simulink model "FOPIDSOCOptimRand"  (R2019b)
settings: Solver=FixedStepAuto  StartTime=0.0  StopTime=30000  FixedStep=0.01  RelTol=1e-3
values from neighbouring files (symbols this model uses):
  L = 10    [benchmarkFOPIDStartReal.m]    (also in benchmarkFOPIStartRealIOLoopL01FOG.m = 0.1; benchmarkFOPIStartRealIOLoopL10FOG.m; benchmarkFOPIStartRealIOLoopL1FOG.m = 1)
  lambdaO = 0.8    [benchmarkFOPIStartRealIOLoopL01FOG.m]
  maxKi = 0.1    [benchmarkFOPIDStartReal.m]    (also in benchmarkFOPIStartRealIOLoopL01FOG.m = 1; benchmarkFOPIStartRealIOLoopL10FOG.m = 0.6; benchmarkFOPIStartRealIOLoopL1FOG.m = 1)
  maxKp = 0.1    [benchmarkFOPIDStartReal.m]    (also in benchmarkFOPIStartRealIOLoopL01FOG.m = 3; benchmarkFOPIStartRealIOLoopL10FOG.m = 2; benchmarkFOPIStartRealIOLoopL1FOG.m = 2)
  minKi = 0.001    [benchmarkFOPIDStartReal.m]    (also in benchmarkFOPIStartRealIOLoopL01FOG.m = 0.3; benchmarkFOPIStartRealIOLoopL10FOG.m = 0.2; benchmarkFOPIStartRealIOLoopL1FOG.m = 0.3)
  minKp = 0.01    [benchmarkFOPIDStartReal.m]    (also in benchmarkFOPIStartRealIOLoopL01FOG.m = 0.3; benchmarkFOPIStartRealIOLoopL10FOG.m = 0.3; benchmarkFOPIStartRealIOLoopL1FOG.m = 0.3)
  ts = 0.01    [benchmarkFOPIStartRealIOLoopL01FOG.m]    (also in benchmarkFOPIStartRealIOLoopL10FOG.m; benchmarkFOPIStartRealIOLoopL1FOG.m; settlingTime.m = time(end))
libraries: dspmathops x1
settings Model: Creator=jairo  LastModifiedBy=jairo
settings DataIOCC: ReturnWorkspaceOutputs=off
settings DebuggingCC: ArithmeticOperatorsInVariantConditions=warning
settings SFSimCC: CustomCodeUndefinedFunction=UseInterfaceOnly

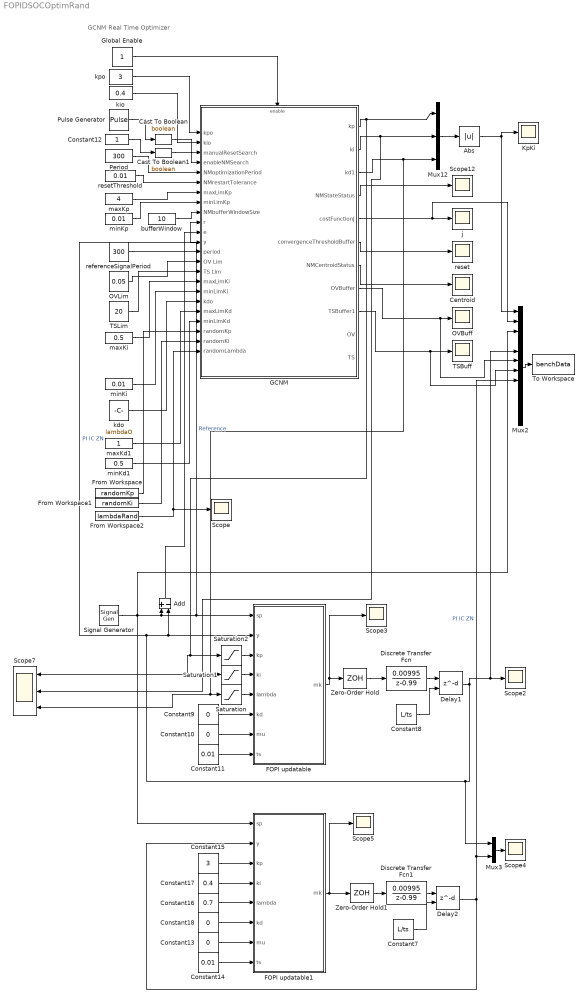
== system FOPIDSOCOptimRand ==
  note: GCNM Real Time Optimizer
  Abs : Abs
  Add : Sum  Inputs=+-
  Cast To Boolean : DataTypeConversion  OutDataTypeStr=boolean
  Cast To Boolean1 : DataTypeConversion  OutDataTypeStr=boolean
  Centroid : Scope
  Constant{9..10,13,18} (4 alike) : Constant  Value=0
  Constant11 : Constant  Value=0.01
  Constant12 : Constant  OutDataTypeStr=boolean
  Constant14 : Constant  Value=0.01
  Constant15 : Constant  Value=3
  Constant16 : Constant  Value=0.7
  Constant17 : Constant  Value=0.4
  Constant7 : Constant  Value=L/ts
  Constant8 : Constant  Value=L/ts
  Delay1 : Delay  DelayLengthSource=Input port
      settings: InputPortMap=u0,p1
  Delay2 : Delay  DelayLengthSource=Input port
      settings: InputPortMap=u0,p1
  Discrete Transfer Fcn : DiscreteTransferFcn  Numerator=[0.00995]  Denominator=[1 -0.99]
  Discrete Transfer Fcn1 : DiscreteTransferFcn  Numerator=[0.00995]  Denominator=[1 -0.99]
  FOPI updatable : Stateflow chart  TreatAsAtomicUnit=on
  FOPI updatable1 : Stateflow chart  TreatAsAtomicUnit=on
  From Workspace : FromWorkspace  VariableName=randomKp  SampleTime=0
  From Workspace1 : FromWorkspace  VariableName=randomKi  SampleTime=0
  From Workspace2 : FromWorkspace  VariableName=lambdaRand  SampleTime=0
  GCNM : Subsystem
  Global Enable : Constant
  KpKi : Scope
  Mux12 : Mux  Inputs=3
  Mux2 : Mux  Inputs=12
  Mux3 : Mux  Inputs=2
  OVBuff : Scope
  OVLim : Constant  Value=0.05
  Period : Constant  Value=300  OutDataTypeStr=double
  Pulse Generator : DiscretePulseGenerator  PulseType=Time based  Period=20  PulseWidth=0.1
  Saturation : Saturate  UpperLimit=1  LowerLimit=0.7
  Saturation1 : Saturate  UpperLimit=maxKi  LowerLimit=minKi
  Saturation2 : Saturate  UpperLimit=maxKp  LowerLimit=minKp
  Scope{,2..5,12} (6 alike) : Scope
  Scope7 : Scope  NumInputPorts=3
  Signal Generator : SignalGenerator  WaveForm=square  Frequency=1/300
  TSBuff : Scope
  TSLim : Constant  Value=20
  To Workspace : ToWorkspace  VariableName=benchData  SaveFormat=Timeseries  SampleTime=-1
  Zero-Order Hold : ZeroOrderHold  SampleTime=-1
  Zero-Order Hold1 : ZeroOrderHold  SampleTime=-1
  bufferWindow : Constant  Value=10  OutDataTypeStr=uint16
  j : Scope
  kdo : Constant  Value=lambdaO
  kio : Constant  Value=0.4  OutDataTypeStr=double
  kpo : Constant  Value=3  OutDataTypeStr=double
  maxKd1 : Constant  VectorParams1D=off  OutDataTypeStr=double
  maxKi : Constant  Value=0.5  VectorParams1D=off  OutDataTypeStr=double
  maxKp : Constant  Value=4  OutDataTypeStr=double
  minKd1 : Constant  Value=0.5  OutDataTypeStr=double
  minKi : Constant  Value=0.01  OutDataTypeStr=double
  minKp : Constant  Value=0.01  OutDataTypeStr=double
  referenceSignalPeriod : Constant  Value=300
  reset : Scope
  resetThreshold : Constant  Value=0.01
  wires:
  FOPI updatable/1(mk) -> Scope3/1, Zero-Order Hold/1
  Discrete Transfer Fcn/1 -> Delay1/1
  Constant9/1 -> FOPI updatable/6(kd)
  Constant11/1 -> FOPI updatable/8(ts)
  Constant10/1 -> FOPI updatable/7(mu)
  Delay1/1 -> Mux2/5, Scope2/1, Mux3/1, FOPI updatable/2(y), Add/2, GCNM/12("  y")  "PI IC ZN"
  maxKd1/1 -> GCNM/19(maxLimKd)
  minKd1/1 -> GCNM/20(minLimKd)
  TSLim/1 -> GCNM/15(TS Lim)
  Period/1 -> GCNM/5(NMoptimizationPeriod)
  Mux12/1 -> Abs/1
  minKi/1 -> GCNM/17(minLimKi)
  GCNM/1("  kp") -> Mux12/1, Saturation2/1, Scope7/1
  GCNM/6(convergenceThresholdBuffer) -> reset/1
  Global Enable/1 -> GCNM/Enable
  GCNM/7(NMCentroidStatus) -> Centroid/1
  Cast To Boolean1/1 -> GCNM/4(enableNMSearch)
  Mux2/1 -> To Workspace/1
  GCNM/5(costFunctionJ) -> Mux2/2, j/1
  OVLim/1 -> GCNM/14("  OV Lim")
  referenceSignalPeriod/1 -> GCNM/13("  period")
  kpo/1 -> GCNM/1(kpo)
  kdo/1 -> GCNM/18(kdo)
  maxKp/1 -> GCNM/7(maxLimKp)
  GCNM/3("  kd1") -> Saturation/1, Scope7/3, Mux12/3
  minKp/1 -> GCNM/8(minLimKp)
  GCNM/8(OVBuffer) -> Mux2/6, OVBuff/1
  Constant12/1 -> Cast To Boolean1/1
  Cast To Boolean/1 -> GCNM/3(manualResetSearch)
  maxKi/1 -> GCNM/16(maxLimKi)
  GCNM/4(NMStateStatus) -> Scope12/1
  kio/1 -> GCNM/2(kio)
  bufferWindow/1 -> GCNM/9(NMbufferWindowSize)
  GCNM/9(TSBuffer1) -> Mux2/7, TSBuff/1
  Pulse Generator/1 -> Cast To Boolean/1
  resetThreshold/1 -> GCNM/6(NMrestartTolerance)
  Signal Generator/1 -> Mux2/3, FOPI updatable1/1(sp), GCNM/10("  r"), FOPI updatable/1(sp), Add/1  "Reference"
  Add/1 -> GCNM/11("  e")
  Constant18/1 -> FOPI updatable1/6(kd)
  Constant14/1 -> FOPI updatable1/8(ts)
  Constant13/1 -> FOPI updatable1/7(mu)
  Mux3/1 -> Scope4/1
  Delay2/1 -> Mux2/8, Mux3/2, FOPI updatable1/2(y)  "PI IC ZN"
  FOPI updatable1/1(mk) -> Scope5/1, Zero-Order Hold1/1
  Constant15/1 -> FOPI updatable1/3(kp)
  Constant17/1 -> FOPI updatable1/4(ki)
  Constant16/1 -> FOPI updatable1/5(lambda)
  From Workspace/1 -> GCNM/21(randomKp)
  From Workspace1/1 -> GCNM/22(randomKi)
  From Workspace2/1 -> Scope/1, GCNM/23(randomLambda)
  Zero-Order Hold/1 -> Discrete Transfer Fcn/1
  Abs/1 -> Mux2/1, KpKi/1
  Zero-Order Hold1/1 -> Discrete Transfer Fcn1/1
  Discrete Transfer Fcn1/1 -> Delay2/1
  GCNM/2("  ki") -> Saturation1/1, Scope7/2, Mux12/2
  Saturation/1 -> FOPI updatable/5(lambda)
  Saturation1/1 -> FOPI updatable/4(ki)
  Saturation2/1 -> FOPI updatable/3(kp)
  Constant8/1 -> Delay1/2
  Constant7/1 -> Delay2/2

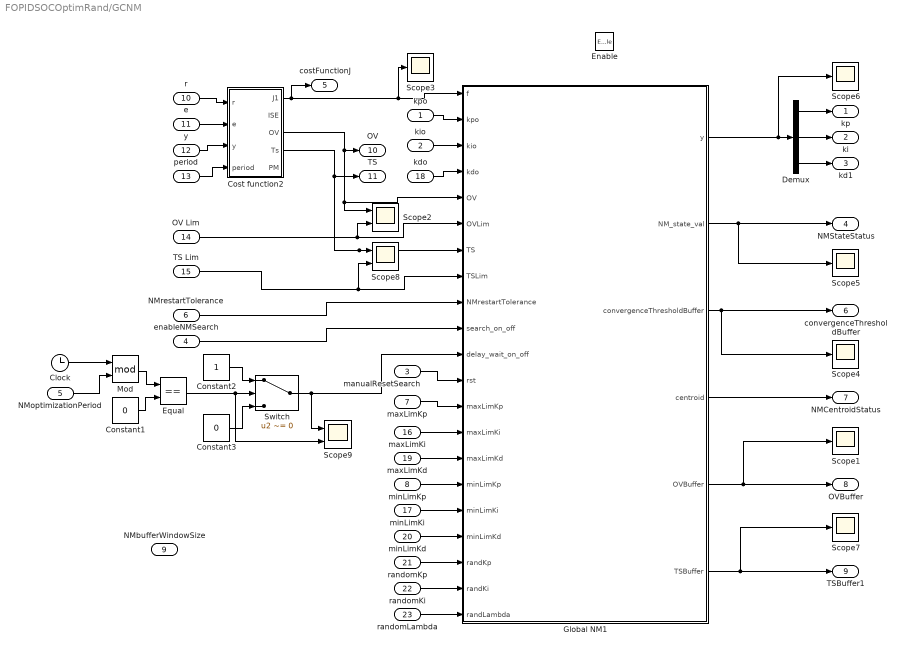
== system FOPIDSOCOptimRand/GCNM ==
  kpo : Inport  OutDataTypeStr=double
  kio : Inport  Port=2  OutDataTypeStr=double
  manualResetSearch : Inport  Port=3  OutDataTypeStr=boolean
  enableNMSearch : Inport  Port=4  OutDataTypeStr=boolean
  NMoptimizationPeriod : Inport  Port=5  OutDataTypeStr=double
  NMrestartTolerance : Inport  Port=6
  maxLimKp : Inport  Port=7  OutDataTypeStr=double
  minLimKp : Inport  Port=8  OutDataTypeStr=double
  NMbufferWindowSize : Inport  Port=9  OutDataTypeStr=uint16
  "  r" : Inport  Port=10  OutDataTypeStr=double
  "  e" : Inport  Port=11  OutDataTypeStr=double
  "  y" : Inport  Port=12  OutDataTypeStr=double
  "  period" : Inport  Port=13  OutDataTypeStr=double
  "  OV Lim" : Inport  Port=14  OutDataTypeStr=double
  TS Lim : Inport  Port=15  OutDataTypeStr=double
  maxLimKi : Inport  Port=16  OutDataTypeStr=double
  minLimKi : Inport  Port=17  OutDataTypeStr=double
  kdo : Inport  Port=18  OutDataTypeStr=double
  maxLimKd : Inport  Port=19  OutDataTypeStr=double
  minLimKd : Inport  Port=20  OutDataTypeStr=double
  randomKp : Inport  Port=21
  randomKi : Inport  Port=22
  randomLambda : Inport  Port=23
  Enable : EnablePort
  Clock : Clock
  Constant1 : Constant  Value=0
  Constant2 : Constant
  Constant3 : Constant  Value=0
  Cost function2 : Subsystem
  Demux : Demux  Outputs=3
  Equal : RelationalOperator  Operator===  RndMeth=Simplest
  Global NM1 : MATLAB Function  TreatAsAtomicUnit=on
  Mod : Math  Operator=mod  SignedPower=off  SaturateOnIntegerOverflow=on
  Scope{1,3..7} (6 alike) : Scope
  Scope2 : Scope  NumInputPorts=2
  Scope8 : Scope  NumInputPorts=2
  Scope9 : Scope  NumInputPorts=2
  Switch : Switch  Criteria=u2 ~= 0
  "  kp" : Outport  OutDataTypeStr=double
  "  ki" : Outport  Port=2  OutDataTypeStr=double
  "  kd1" : Outport  Port=3  OutDataTypeStr=double
  NMStateStatus : Outport  Port=4  OutDataTypeStr=double
  costFunctionJ : Outport  Port=5  OutDataTypeStr=double
  convergenceThresholdBuffer : Outport  Port=6  OutDataTypeStr=double
  NMCentroidStatus : Outport  Port=7  OutDataTypeStr=double
  OVBuffer : Outport  Port=8  OutDataTypeStr=double
  TSBuffer1 : Outport  Port=9  OutDataTypeStr=double
  OV : Outport  Port=10  OutDataTypeStr=double
  TS : Outport  Port=11  OutDataTypeStr=double
  wires:
  Demux/2 -> "  ki"/1
  Demux/1 -> "  kp"/1
  NMrestartTolerance/1 -> Global NM1/9(NMrestartTolerance)
  manualResetSearch/1 -> Global NM1/12(rst)
  enableNMSearch/1 -> Global NM1/10(search_on_off)
  minLimKp/1 -> Global NM1/16(minLimKp)
  maxLimKp/1 -> Global NM1/13(maxLimKp)
  Global NM1/2(NM_state_val) -> NMStateStatus/1, Scope5/1
  Global NM1/3(convergenceThresholdBuffer) -> convergenceThresholdBuffer/1, Scope4/1
  Global NM1/4(centroid) -> NMCentroidStatus/1
  Global NM1/1(y) -> Scope6/1, Demux/1
  kpo/1 -> Global NM1/2(kpo)
  kio/1 -> Global NM1/3(kio)
  Cost function2/3(OV) -> OV/1, Global NM1/5(OV), Scope2/1
  "  y"/1 -> Cost function2/3(y)
  "  e"/1 -> Cost function2/2(e)
  "  r"/1 -> Cost function2/1(r)
  Global NM1/5(OVBuffer) -> Scope1/1, OVBuffer/1
  "  period"/1 -> Cost function2/4(period)
  "  OV Lim"/1 -> Scope2/2, Global NM1/6(OVLim)
  Cost function2/4(Ts) -> TS/1, Global NM1/7(TS), Scope8/1
  TS Lim/1 -> Scope8/2, Global NM1/8(TSLim)
  Global NM1/6(TSBuffer) -> Scope7/1, TSBuffer1/1
  Cost function2/1(J1) -> Scope3/1, Global NM1/1(f), costFunctionJ/1
  Clock/1 -> Mod/1
  NMoptimizationPeriod/1 -> Mod/2
  Constant1/1 -> Equal/2
  Mod/1 -> Equal/1
  Constant2/1 -> Switch/1
  Constant3/1 -> Switch/3
  Switch/1 -> Scope9/1, Global NM1/11(delay_wait_on_off)
  Equal/1 -> Scope9/2, Switch/2
  maxLimKi/1 -> Global NM1/14(maxLimKi)
  minLimKi/1 -> Global NM1/17(minLimKi)
  kdo/1 -> Global NM1/4(kdo)
  maxLimKd/1 -> Global NM1/15(maxLimKd)
  minLimKd/1 -> Global NM1/18(minLimKd)
  randomKp/1 -> Global NM1/19(randKp)
  randomKi/1 -> Global NM1/20(randKi)
  randomLambda/1 -> Global NM1/21(randLambda)
  Demux/3 -> "  kd1"/1

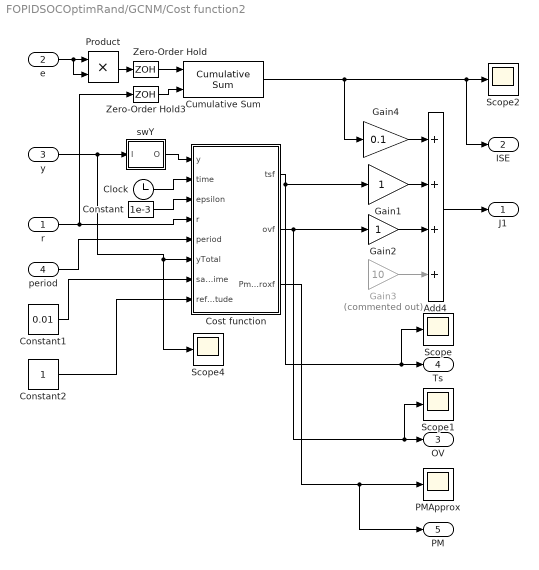
== system FOPIDSOCOptimRand/GCNM/Cost function2 ==
  r : Inport
  e : Inport  Port=2
  y : Inport  Port=3
  period : Inport  Port=4
  Add4 : Sum  Inputs=++++
  Clock : Clock
  Constant : Constant  Value=1e-3
  Constant1 : Constant  Value=0.01
  Constant2 : Constant
  Cost function : MATLAB Function  TreatAsAtomicUnit=on
  Cumulative Sum : dspmathops/Cumulative Sum  dim=Channels (running sum)  InputProcessing=Columns as channels (frame based)  reset_popup=Falling edge  roundingMode=Floor  overflowMode=off  outputDataTypeStr=Inherit: Same as accumulator  outputMin=[]  outputMax=[]  outputLastDataTypeStr=Inherit: Same as accumulator
      settings: SourceProductName=DSP System Toolbox
  Gain1 : Gain
  Gain2 : Gain
  Gain3 : Gain  Commented=on  Gain=10
  Gain4 : Gain  Gain=0.1
  PMApprox : Scope
  Product : Product
  Scope{,1..2,4} (4 alike) : Scope
  Zero-Order Hold : ZeroOrderHold  SampleTime=-1
  Zero-Order Hold3 : ZeroOrderHold  SampleTime=-1
  swY : Subsystem
  J1 : Outport
  ISE : Outport  Port=2
  OV : Outport  Port=3
  Ts : Outport  Port=4
  PM : Outport  Port=5
  wires:
  Cumulative Sum/1 -> Gain4/1, ISE/1, Scope2/1
  Zero-Order Hold3/1 -> Cumulative Sum/2
  e/1 -> Product/2, Product/1
  Zero-Order Hold/1 -> Cumulative Sum/1
  r/1 -> Zero-Order Hold3/1, Cost function/4(r)
  swY/1(O) -> Cost function/1(y)
  Clock/1 -> Cost function/2(time)
  Product/1 -> Zero-Order Hold/1
  Constant/1 -> Cost function/3(epsilon)
  y/1 -> Scope4/1, Cost function/6(yTotal), swY/1(I)
  Add4/1 -> J1/1
  Gain2/1 -> Add4/3
  period/1 -> Cost function/5(period)
  Constant1/1 -> Cost function/7(samplingTime)
  Gain1/1 -> Add4/2
  Constant2/1 -> Cost function/8(refAmplitude)
  Gain3/1 -> Add4/4
  Cost function/1(tsf) -> Scope/1, Ts/1, Gain1/1
  Cost function/2(ovf) -> Scope1/1, OV/1, Gain2/1
  Cost function/3(PmAproxf) -> PM/1, PMApprox/1
  Gain4/1 -> Add4/1

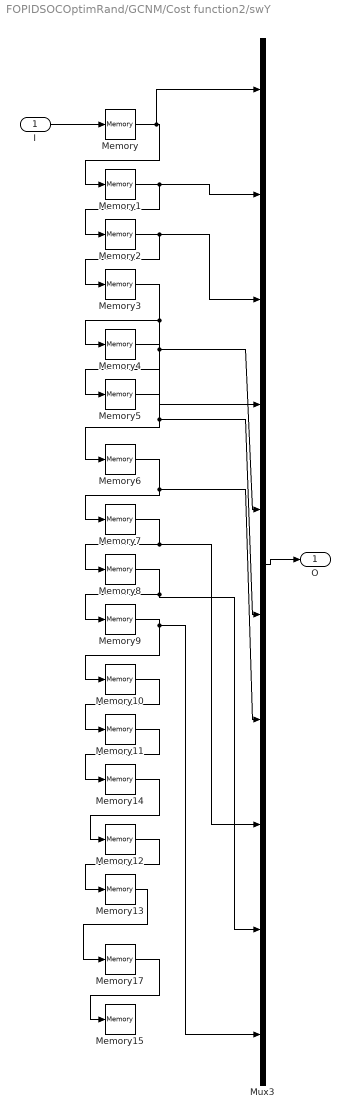
== system FOPIDSOCOptimRand/GCNM/Cost function2/swY ==
  I : Inport
  Memory{,1..15,17} (17 alike) : Memory
  Mux3 : Mux  Inputs=10
  O : Outport
  wires:
  Memory11/1 -> Memory14/1
  Memory14/1 -> Memory12/1
  Memory12/1 -> Memory13/1
  Memory13/1 -> Memory17/1
  Memory5/1 -> Memory6/1, Mux3/6
  Memory4/1 -> Memory5/1, Mux3/5
  Mux3/1 -> O/1
  Memory9/1 -> Memory10/1, Mux3/10
  Memory3/1 -> Memory4/1, Mux3/4
  Memory6/1 -> Memory7/1, Mux3/7
  Memory1/1 -> Memory2/1, Mux3/2
  Memory10/1 -> Memory11/1
  Memory2/1 -> Memory3/1, Mux3/3
  I/1 -> Memory/1
  Memory8/1 -> Memory9/1, Mux3/9
  Memory/1 -> Memory1/1, Mux3/1
  Memory7/1 -> Memory8/1, Mux3/8
  Memory17/1 -> Memory15/1

== stateflow chart FOPIDSOCOptimRand/FOPI updatable ==
  settings: updateMethod=DISCRETE  sampleTime=0.01
  state control
    %gains calculation at each control step
    ti=kp/ki;
    td=kd/kp;
    Tt=sqrt(td*ti);    %antiwindup calculation
    %lambda_1=lambda;  %adjusting of integral order
    lambda_1=1-lambda;  %adjusting of integral order
    alfa=wc/tan(wc*(ts/2));
    alfa_lambda=alfa^lambda;   %este es el lambda orignal
    a5=-2*lambda_1;
    a4=-2*(lambda_1^2);
    a3=-( ((4/3)*lambda_1^3) + ((2/3)*lambda_1)  );
    a2=( ((2/3)*lambda_1^4) + ((4/3)*lambda_1^2)  );
    a1=-( ((4/15)*lambda_1^5) + ((4/3)*lambda_1^3) + ((2/5)*lambda_1) );
    a0=-( ((4/45)*lambda_1^6) + ((8/9)*lambda_1^4) + ((46/45)*lambda_1^2) );
    r=ki/alfa_lambda;
    alfa_mu=alfa^mu;
    b5=-2*mu;
    b4=-2*(mu^2);
    b3=-( ((4/3)*mu^3) + ((2/3)*mu)  );
    b2=( ((2/3)*mu^4) + ((4/3)*mu^2)  );
    b1=-( ((4/15)*mu^5) + ((4/3)*mu^3) + ((2/5)*mu) );
    b0=-( ((4/45)*mu^6) + ((8/9)*mu^4) + ((46/45)*mu^2) );
    r1=kd*alfa_mu;
    %FOPI controller calculation
    entry: ek=sp-y;
    mkp=kp*ek;
    mki= (r*(ek+ek_1)) - ((a5-1)*mki_1) - ((a4-a5)*mki_2) - ( (a3-a4)*mki_3 ) - ( (a2-a3)*mki_4 )- ( (a1-a2)*mki_5 ) - ( (a0-a1)*mki_6 )+( (a0)*mki_7);
    //mkd=r1*(  (ek)-(b5*ek_1)+(b4*ek_2)+(b3*ek_3)+(b2*ek_4)+(b1*ek_5)+(b0*ek_6) );
    //mka=mkp+mki+mkd;
    mka=mkp+mki;
  state inicio
    %constantes FOPID
    entry:
    mk_sat_pos=255;
    mk_sat_neg=-255;
    ek_1=0;ek_2=0; ek_3=0; ek_4=0; ek_5=0; ek_6=0;
    mki_1=0; mki_2=0; mki_3=0; mki_4=0; mki_5=0; mki_6=0; mki_7=0;
    %constantes
    wc=10;                        %gain crossover frequency
  (default) -> inicio
  control -> (junction 4)
  inicio -> control
  (junction 4) -> (junction 7) [order 1] : [mka>mk_sat_pos]
  (junction 4) -> (junction 6) [order 2]
  (junction 7) -> (junction 8) : {mki=mki-(1/Tt)*(mka-mk_sat_pos); mka=mk_sat_pos;}
  (junction 6) -> (junction 9) [order 1] : [mka<mk_sat_neg]
  (junction 6) -> (junction 5) [order 2]
  (junction 9) -> (junction 10) : {mki=mki-(1/Tt)*(mka-mk_sat_neg);mka=mk_sat_neg;}
  (junction 10) -> (junction 5)
  (junction 8) -> (junction 10)
  (junction 5) -> (junction 11)
  (junction 11) -> control : {mki_7=mki_6;
      | mki_6=mki_5;
      | mki_5=mki_4;
      | mki_4=mki_3;
      | mki_3=mki_2;
      | mki_2=mki_1;
      | mki_1=mki;
      | ek_6=ek_5; ek_5=ek_4;
      | ek_4=ek_3; ek_3=ek_2;
      | ek_2=ek_1; ek_1=ek;
      | mk=mka}
  data: mkd local double; Tt local double; mk_sat_pos local double; mk_sat_neg local double; ek_1 local double; mki_1 local double; ek local double; mkp local double; mki local double; mk output double; sp input; y input; mka local double; r1 local double; r2 local double; ek_2 local double; mki_2 local double; a0 local double; a1 local double; a2 local double; a3 local double; a4 local double; a5 local double; alfa local double; alfa_lambda local double; lambda_1 local double; mki_3 local double; mki_4 local double; mki_5 local double; mki_6 local double; mki_7 local double; r local double; wc local double; b0 local double; b1 local double; b2 local double; b3 local double; b4 local double; b5 local double; ek_3 local double; ek_4 local double; ek_5 local double; ek_6 local double; alfa_mu local double; kp input double; ki input double; lambda input double; ti local double; td local double; kd input double; mu input double; ts input double

== matlab function FOPIDSOCOptimRand/GCNM/Global NM1 ==
  settings: updateMethod=DISCRETE
  data: f input; y output size=3; kpo input; kio input; kdo input; OV input; OVLim input; TS input; TSLim input; NM_state_val output; convergenceThresholdBuffer output; NMrestartTolerance input; centroid output; search_on_off input; delay_wait_on_off input; rst input; OVBuffer output; maxLimKp input; maxLimKi input; maxLimKd input; minLimKp input; TSBuffer output; minLimKi input; minLimKd input; randKp input; randKi input; randLambda input
%function [y, NM_state_val,convergenceThresholdBuffer,centroid,BiasRFState1ReflectionCoefficientBuffer]= fcn(f,kpo, kio,BiasRFState1ReflectionCoefficient,BiasRFState1ReflectionCoefficientLim,...
%                                                                                                            NMrestartTolerance, search_on_off, delay_wait_on_off, rst,maxLim,minLim)
function [y, NM_state_val,convergenceThresholdBuffer,centroid,OVBuffer,TSBuffer]= fcn(f,kpo, kio,kdo,OV,OVLim,TS,TSLim,...
                                                                                                           NMrestartTolerance, search_on_off, delay_wait_on_off, rst,maxLimKp,maxLimKi,maxLimKd,minLimKp,minLimKi,minLimKd,randKp,randKi,randLambda)

% persistent count
persistent NM_state         %Integer definition for states, since enum is not supported
persistent Full_eval_count
persistent usual_delta      %5 percent deltas for non-zero terms
persistent zero_term_delta  %Even smaller delta for zero elements of x
persistent v fv v_r v_e v_m f_r v_c 
persistent yp               %last output when search was on
persistent delay_edge
persistent delay_wait_on_off_z
persistent f_old
persistent windowCounter convergenceThresholdStd gamma1Std gamma2Std delta1Std  ps1Std ps2Std delta2Std
persistent bufferJ bufferGamma1 bufferGamma2 bufferDelta1 bufferDelta2 bufferPS1 bufferPS2;

x=[kpo,kio,kdo];  %Initial conditions vector for kp and ki terms

%mead algorithm reset using normal distribution with 1000 choices of initial conditions for Nelder
n = 3;      %Input dimension - needs to be defined as a constant to keep Simulink port width inheretence happy
np1 = n+1;  %Simplex solid dimension
n_r = 1/n;  %Calculate reciprocal at compilation time for mean calculation

%Simplex update coefficients %Can be a function of dimension see Han2010
% alpha = 1;
% beta = 2;
% gamma = 0.5;
% delta = 0.5;

%Adaptive simplex search coefficients: Han2010
alpha = 1;%0.5;
beta = 1 + 2*n_r;%0.5 + 2*n_r;
gamma = 0.75 - 0.5*n_r;
% delta = 1 - n_r;
delta=0;


bufferWindow=10;
%NM_state:  
    %0 - Initial   (Initialize vertices)
    %1 - FVE: Full vertex evaluation (with insertion sort after each evaluation)
    %2 - Insertion Sort (After Reflection, Expansion or Contraction Steps)
    %3 - Reflection Entry
    %4 - Reflection Evaluate
    %5 - Expansion
    %6 - Outside Contraction
    %7 - Inside Contraction
    %(8) - Shrink (Implicit on contraction outcome)

%Full_eval_count:
    %Number of initial vertices evaluated
    xin = x(:);         %Force xin to be a column vector
    coder.cinclude('<time.h>')   %% add the library time.c to the generated code
%initialization state of the Nelder Mead
    if isempty(NM_state)
        
        sd=0;
        sd=coder.ceval('time',[]);   %take the seed from the system current time
        rng(sd,'twister');           %initialize the seed of the system using current system seed

        delay_edge = 0;
        yp = xin;
        delay_wait_on_off_z = 0;
        convergenceThresholdStd=100;
        gamma1Std=1;
        gamma2Std=1;
        delta1Std=1;
        delta2Std=1;
        ps1Std=1;
        ps2Std=1;

        windowCounter=1; 
        bufferJ=zeros(1,bufferWindow);
        bufferGamma1=zeros(1,bufferWindow); 
        bufferGamma2=zeros(1,bufferWindow);
        bufferDelta1=zeros(1,bufferWindow); 
        bufferDelta2=zeros(1,bufferWindow); 
        bufferPS1=zeros(1,bufferWindow);
        bufferPS2=zeros(1,bufferWindow);
        
        v = zeros(n,np1);   %Initialize n+1 vertices for simplex
        fv = zeros(1,np1);  %function values at the vertices
        v_m = v(:,1);       %0 vector
        v_r = v_m;          %0 vector    
        v_e = v_m;          %0 vector
        v_c = v_m;          %0 vector
        f_r = 0;          %0 vector

%         usual_delta = 0.01; %original 0.07
        usual_delta = 0.1; %original 0.07
%         zero_term_delta = 0.000025;
        zero_term_delta = 0.0025;
        NM_state = 0;          %Initial state
        Full_eval_count = 1;   %No vertices evaulated, yet

        v(:,1) = xin;
        for j=1:n
            vt = xin;
            if vt(j) ~= 0
                vt(j) = (1 + usual_delta)*vt(j);
            else
                vt(j) = zero_term_delta;
            end
            v(:, j+1) = vt;
        end
        v(2,:)=v(2,:);
    end
    
    
% if (rst==1)  %%Reset the search (Forced reset by external source)
%         f_old = 0;
%         delay_edge = 0;
%         y = xin;
%         delay_wait_on_off_z = 0;
%         convergenceThresholdStd=0;
%        
%         windowCounter=1; 
%         bufferJ=zeros(1,bufferWindow);
%         bufferGamma1=zeros(1,bufferWindow); 
%         bufferGamma2=zeros(1,bufferWindow);
%         bufferDelta1=zeros(1,bufferWindow); 
%         bufferDelta2=zeros(1,bufferWindow); 
%         bufferPS1=zeros(1,bufferWindow);
%         bufferPS2=zeros(1,bufferWindow);
%         
%         v = zeros(n,np1);   %Initialize n+1 vertices for simplex
%         fv = zeros(1,np1);  %function values at the vertices
%         v_m = v(:,1);       %0 vector
%         v_r = v_m;          %0 vector    
%         v_e = v_m;          %0 vector
%         v_c = v_m;          %0 vector
%         f_r = 0;          %0 vector
% 
%         usual_delta = 0.05;
%         zero_term_delta = 0.00025;
%         
% %         usual_delta = 0.1; %Use for force cross decoupling search
% %         zero_term_delta = 0.05; %Use for force cross decoupling search
% 
%         NM_state = 0;          %Initial state
%         Full_eval_count = 1;   %No vertices evaulated, yet
% 
%         v(:,1) = xin;
%         
%         for j=1:n
%             vt = xin;
%             if vt(j) ~= 0
%                 vt(j) = (1 + usual_delta)*vt(j);
%             else
%                 vt(j) = zero_term_delta;
%             end
%             v(:, j+1) = vt;
%         end
% end



%+++++++++++++ NM search enabling rising flank+++++++++++++++++++++++++++++
% if ((delay_wait_on_off_z == 1) && (delay_wait_on_off == 0))  %falling edge detection for delay_wait_on_off
if ((delay_wait_on_off_z == 0) && (delay_wait_on_off == 1)) %rising edge detection for delay_wait_on_off
    delay_edge = 1;    
    elseif ((delay_wait_on_off_z == 0) && (delay_wait_on_off == 0)) %while level is low
% elseif ((delay_wait_on_off_z == 1) && (delay_wait_on_off == 1)) %while level is high
    delay_edge = 0;
end
    
   
    
%%%++++++++++NM optimization algorithm execution if enable and rising flank are activated   
if ((search_on_off==1) && (delay_edge==1))  




    %restart initialization routine
    gammaCond=(gamma1Std>=OVLim );%|| gamma2Std>=BiasRFState2ReflectionCoefficientLim);
    deltaCond=(gamma2Std>=TSLim);% || delta2Std>=ADVCIPowerSetpointState2Lim);
%     psCond=(ps1Std>=ADVCIPulseQualityDeviationState1Lim || ps2Std>=ADVCIPulseQualityDeviationState2Lim);
    if (abs(convergenceThresholdStd)<= NMrestartTolerance && (gammaCond==1) || deltaCond==1)% || psCond==1) )%&& v_m(1,:)~=0)   %fv(1)>-28       %redo void case, restart the search

           v = zeros(n,np1);   %Initialize n+1 vertices for simplex
           fv = zeros(1,np1);      %function values at the vertices
            v_m = v(:,1);       %0 vector
            v_r = v_m;          %0 vector    
            v_e = v_m;          %0 vector
            v_c = v_m;          %0 vector
            f_r = 0;            %0 vector

%             usual_delta = 0.005;
            usual_delta = 0.01;
            zero_term_delta = 0.025;
            NM_state = 0;          %Initial state
            Full_eval_count = 1;   %No vertices evaulated, yet

%             %new initial condition for probabilistic restart
% %             v(:,1) = (maxLim*rand(2,1));
%             v(1,1) = (maxLimKp*rand(1,1));
%             v(2,1) = (maxLimKi*rand(1,1));
%             v(3,1) = (maxLimKi*rand(1,1));
%             while ((v(1,1)>maxLimKp || v(1,1)<minLimKp) || (v(2,1)>maxLimKi || v(2,1)<minLimKi) || (v(3,1)>maxLimKd || v(3,1)<minLimKd))==1
%                 v(1,1) = (maxLimKp*rand(1,1));
%                 v(2,1) = (maxLimKi*rand(1,1));
%                 v(3,1) = (maxLimKd*rand(1,1));
%                 v(:,1);
%             end
            %new initial condition generated outside the block
            xin=[randKp;randKi;randLambda];



            v(:,1)=xin;

            for j=1:n
                vt = xin;
                if vt(j) ~= 0
                    vt(j) = (1 + usual_delta)*vt(j);
                else
                    vt(j) = zero_term_delta;
                end
                v(:, j+1) = vt;
            end   
        convergenceThresholdStd=1;


    end    


    %%%%%%%%%%%%%%%%%%%%%% Nelder Mead State selection  %%%%%%%%%%%%%%%%%%%%%%%     
        switch NM_state  
            case 0 %Vertices has just been initialized
              y = v(:, Full_eval_count); %Write out first vertex for evaluation
              NM_state = 1;

            case 1 %Full vertex evaluation  
                fv(Full_eval_count) = f; %costFunctionJ;  %Read evaluated function value

                j = Full_eval_count;  %New value came in, insert it into sorted list
                while ( (j>1) && (fv(j-1)>fv(j)) ) %Sort ascending
                   temp = fv(j-1);
                   fv(j-1) = fv(j);
                   fv(j) = temp;
                   temp = v(:, j-1);
                   v(:, j-1) = v(:, j); %Also sort corresponding (evaluated) vertices 
                   v(:, j) = temp;
                   j = j-1;
                end

                Full_eval_count = Full_eval_count + 1;            
                if (Full_eval_count <= (np1))
                    y = v(:, Full_eval_count);                
                else
                    Full_eval_count = Full_eval_count - 1; 
                    %NM_state = 3;   %Full vertex evaluation complete -> Reflection 
                    v_sum = xin*0;  %Initialize sum for mean calculation

                    for i=1:n
                        v_sum = v_sum + v(:, i);
                    end

                    v_m = v_sum*n_r; %Centroid
                    v_r  = v_m*(1+alpha) - alpha*v(:, end);
                    y  = v_r;
                    NM_state = 4;   %Reflection Evaluate
                end

            case 2 %Insertion Sort                        
                    j = Full_eval_count;  %New value came in, insert it into list
                       while ( (j>1) && (fv(j-1)>fv(j)) ) %Sort ascending
                           temp = fv(j-1);
                           fv(j-1) = fv(j);
                           fv(j) = temp;
                           temp = v(:, j-1);
                           v(:, j-1) = v(:, j); %Also sort corresponding (evaluated) vertices 
                           v(:, j) = temp;
                           j = j-1;
                       end
                       y  = v_r;
                    NM_state = 3;   %Reflection 

            case 3 %Reflection Entry
                    v_sum = xin*0;  %Initialize sum for mean calculation

                    for i=1:n
                        v_sum = v_sum + v(:, i);
                    end

                    v_m = v_sum*n_r; %Centroid
                    v_r  = v_m*(1+alpha) - alpha*v(:, np1);
                    y  = v_r;
                    NM_state = 4;   %Reflection Evaluate

            case 4 %Reflection Evaluate
                f_r = f; %costFunctionJ;
                if ( (f_r>fv(:, 1)) && (f_r<fv(:, n)) )
                    v(:, np1) = v_r;
                    fv(np1) = f_r;
                    %NM_state = 2;
                    j = Full_eval_count;  %New value came in, insert it into list
                    while ( (j>1) && (fv(j-1)>fv(j)) ) %Sort ascending
                       temp = fv(j-1);
                       fv(j-1) = fv(j);
                       fv(j) = temp;
                       temp = v(:, j-1);
                       v(:, j-1) = v(:, j); %Also sort corresponding (evaluated) vertices 
                       v(:, j) = temp;
                       j = j-1;
                    end
                    %%NM_state = 3;   %Reflection 

                    v_sum = xin*0;  %Initialize sum for mean calculation

                    for i=1:n
                        v_sum = v_sum + v(:, i);
                    end

                    v_m = v_sum*n_r; %Centroid
                    v_r  = v_m*(1+alpha) - alpha*v(:, np1);
                    y  = v_r;
                    NM_state = 4;    %Reflection Evaluate
                elseif (f_r<fv(:, 1))
                    v_e  = v_m*(1-beta) + beta*v_r; 
                    y  = v_e;
                    NM_state = 5;    %Expansion
                else
                    if ( (f_r>=fv(n)) && (f_r<fv(np1)) ) 
                        v_c  = v_m*(1-gamma) + gamma*v_r; 
                        NM_state = 6; %Outside Contraction
                    elseif (f_r>=fv(np1))  
                        v_c  = v_m*(1+gamma) - gamma*v_r; 
                        NM_state = 7; %Inside Contraction
                    end
                    y = v_c;
                end

            case 5 %Expansion
                f_e = f; %costFunctionJ;
                if (f_e<f_r)
                    v(:, end) = v_e;
                    fv(end) = f_e;
                    %NM_state = 2;
                        j = Full_eval_count;  %New value came in, insert it into list
                       while ( (j>1) && (fv(j-1)>fv(j)) ) %Sort ascending
                           temp = fv(j-1);
                           fv(j-1) = fv(j);
                           fv(j) = temp;
                           temp = v(:, j-1);
                           v(:, j-1) = v(:, j); %Also sort corresponding (evaluated) vertices 
                           v(:, j) = temp;
                           j = j-1;
                       end
                    %%NM_state = 3;   %Reflection 

                    v_sum = xin*0;  %Initialize sum for mean calculation

                    for i=1:n
                        v_sum = v_sum + v(:, i);
                    end

                    v_m = v_sum*n_r; %Centroid
                    v_r  = v_m*(1+alpha) - alpha*v(:, np1);
                    y  = v_r;
                    NM_state = 4;   %Reflection Evaluate
                 else
                    v(:, np1) = v_r;
                    fv(np1) = f_r;
                    %NM_state = 2;
                    j = Full_eval_count;  %New value came in, insert it into list
                   while ( (j>1) && (fv(j-1)>fv(j)) ) %Sort ascending
                       temp = fv(j-1);
                       fv(j-1) = fv(j);
                       fv(j) = temp;
                       temp = v(:, j-1);
                       v(:, j-1) = v(:, j); %Also sort corresponding (evaluated) vertices 
                       v(:, j) = temp;
                       j = j-1;
                   end

                   %%NM_state = 3;   %Reflection 

                    v_sum = xin*0;  %Initialize sum for mean calculation

                    for i=1:n
                        v_sum = v_sum + v(:, i);
                    end

                    v_m = v_sum*n_r; %Centroid
                    v_r  = v_m*(1+alpha) - alpha*v(:, np1);
                    y  = v_r;
                    NM_state = 4;   %Reflection Evaluate
                end

           case 6 %Contraction
               f_c = f;%costFunctionJ;
               if (f_c<f_r)
                   v(:, np1) = v_c;
                   fv(np1) = f_c;
                   %NM_state = 2;
                   j = Full_eval_count;  %New value came in, insert it into list
                   while ( (j>1) && (fv(j-1)>fv(j)) ) %Sort ascending
                       temp = fv(j-1);
                       fv(j-1) = fv(j);
                       fv(j) = temp;
                       temp = v(:, j-1);
                       v(:, j-1) = v(:, j); %Also sort corresponding (evaluated) vertices 
                       v(:, j) = temp;
                       j = j-1;
                   end
                    %%NM_state = 3;   %Reflection 

                    v_sum = xin*0;  %Initialize sum for mean calculation

                    for i=1:n
                        v_sum = v_sum + v(:, i);
                    end

                    v_m = v_sum*n_r; %Centroid
                    v_r  = v_m*(1+alpha) - alpha*v(:, np1);
                    y  = v_r;
                    NM_state = 4;   %Reflection Evaluate
               else
                   for j=2:n+1   %Shrink
                     v(:,j) = v(:,1)*(1-delta) + delta*v(:,j);
                   end
                   y = v(:, 2);   %Start with evaluation
                   Full_eval_count = 2; 
                   NM_state = 1; %Full vertex evaluation after shrink
               end
            case 7
                f_c = f;%costFunctionJ;
                   if (f_c<fv(np1))
                       v(:, np1) = v_c;
                       fv(np1) = f_c;
                       %NM_state = 2;
                        j = Full_eval_count;  %New value came in, insert it into list
                        while ( (j>1) && (fv(j-1)>fv(j)) ) %Sort ascending
                           temp = fv(j-1);
                           fv(j-1) = fv(j);
                           fv(j) = temp;
                           temp = v(:, j-1);
                           v(:, j-1) = v(:, j); %Also sort corresponding (evaluated) vertices 
                           v(:, j) = temp;
                           j = j-1;
                        end
                        NM_state = 3;   %Reflection 

                        v_sum = xin*0;  %Initialize sum for mean calculation

                        for i=1:n
                            v_sum = v_sum + v(:, i);
                        end

                        v_m = v_sum*n_r; %Centroid
                        v_r  = v_m*(1+alpha) - alpha*v(:, np1);
                        y  = v_r;
    %                     NM_state = 4;   %Reflection Evaluate
                   else
                       for j=2:n+1 %Shrink
                         v(:,j) = v(:,1)*(1-delta) + delta*v(:,j);
                       end
                       y = v(:,2);   %Start with evaluation
                       Full_eval_count = 2; 
                       NM_state = 1; %Full vertex evaluation after shrink  
                   end     
            otherwise
            y = v(:,1);
         end %End switch NM_states   

         %restart window implemented inside the GCNM function

        bufferJ(windowCounter)=v_m(1,1);                                    %centroid window instead cost function (working without noise)
        bufferGamma1(windowCounter)=OV;
        bufferGamma2(windowCounter)=TS;
%         bufferDelta1(windowCounter)=BiasRFState1PowerSetpointError;
%         bufferDelta2(windowCounter)=BiasRFState2PowerSetpointError;
%         bufferPS1(windowCounter)=  ADVCIPulseQualityDeviationState1;
%         bufferPS2(windowCounter)=  ADVCIPulseQualityDeviationState2;

    %      bufferJ(windowCounter)=f; %cost function window 
         windowCounter=windowCounter+1;
         if windowCounter>bufferWindow
            convergenceThresholdStd=(std(bufferJ));
            gamma1Std=(mean(bufferGamma1));
            gamma2Std=(mean(bufferGamma2));
            delta1Std=(mean(bufferDelta1));
            delta2Std=(mean(bufferDelta2));
            ps1Std=(mean(bufferPS1));
            ps2Std=(mean(bufferPS2));

            windowCounter=1;

         end


    else            %this condition appears when the controller is disabled
         y = yp;
         gammaCond=true;
         deltaCond=true;
%          psCond=true;
     
end

%outputs definitions
     yp = y;
%      if y(3)<0.7
%          y(3)=0.7;
%      elseif y(3)>1
%          y(3)=1;
%      end
%      
     NM_state_val = NM_state;
     centroid= v_m; 
     delay_wait_on_off_z = delay_wait_on_off; 
     %sliding window updating
     convergenceThresholdBuffer=convergenceThresholdStd;      %std
     %buffers constraint condition update
             
        OVBuffer=gamma1Std;
        TSBuffer=gamma2Std;
%         BiasRFState1PowerSetpointErrorBuffer=delta1Std;
%         BiasRFState2PowerSetpointErrorBuffer=delta2Std;
%         ADVCIPulseQualityDeviationState1Buffer=ps1Std;
%         ADVCIPulseQualityDeviationState2Buffer=ps2Std;
%      
     
     
end %End of function

== stateflow chart FOPIDSOCOptimRand/FOPI updatable1 ==
  settings: updateMethod=DISCRETE  sampleTime=0.01
  state control
    %gains calculation at each control step
    ti=kp/ki;
    td=kd/kp;
    Tt=sqrt(td*ti);    %antiwindup calculation
    lambda_1=1-lambda;  %adjusting of integral order
    alfa=wc/tan(wc*(ts/2));
    alfa_lambda=alfa^lambda;   %este es el lambda orignal
    a5=-2*lambda_1;
    a4=-2*(lambda_1^2);
    a3=-( ((4/3)*lambda_1^3) + ((2/3)*lambda_1)  );
    a2=( ((2/3)*lambda_1^4) + ((4/3)*lambda_1^2)  );
    a1=-( ((4/15)*lambda_1^5) + ((4/3)*lambda_1^3) + ((2/5)*lambda_1) );
    a0=-( ((4/45)*lambda_1^6) + ((8/9)*lambda_1^4) + ((46/45)*lambda_1^2) );
    r=ki/alfa_lambda;
    alfa_mu=alfa^mu;
    b5=-2*mu;
    b4=-2*(mu^2);
    b3=-( ((4/3)*mu^3) + ((2/3)*mu)  );
    b2=( ((2/3)*mu^4) + ((4/3)*mu^2)  );
    b1=-( ((4/15)*mu^5) + ((4/3)*mu^3) + ((2/5)*mu) );
    b0=-( ((4/45)*mu^6) + ((8/9)*mu^4) + ((46/45)*mu^2) );
    r1=kd*alfa_mu;
    %FOPI controller calculation
    entry: ek=sp-y;
    mkp=kp*ek;
    mki= (r*(ek+ek_1)) - ((a5-1)*mki_1) - ((a4-a5)*mki_2) - ( (a3-a4)*mki_3 ) - ( (a2-a3)*mki_4 )- ( (a1-a2)*mki_5 ) - ( (a0-a1)*mki_6 )+( (a0)*mki_7);
    mkd=r1*(  (ek)-(b5*ek_1)+(b4*ek_2)+(b3*ek_3)+(b2*ek_4)+(b1*ek_5)+(b0*ek_6) );
    //mka=mkp+mki+mkd;
    mka=mkp+mki;
  state inicio
    %constantes FOPID
    entry:
    mk_sat_pos=255;
    mk_sat_neg=-255;
    ek_1=0;ek_2=0; ek_3=0; ek_4=0; ek_5=0; ek_6=0;
    mki_1=0; mki_2=0; mki_3=0; mki_4=0; mki_5=0; mki_6=0; mki_7=0;
    %constantes
    wc=1;                        %gain crossover frequency
  (default) -> inicio
  control -> (junction 4)
  inicio -> control
  (junction 4) -> (junction 7) [order 1] : [mka>mk_sat_pos]
  (junction 4) -> (junction 6) [order 2]
  (junction 7) -> (junction 8) : {mki=mki-(1/Tt)*(mka-mk_sat_pos); mka=mk_sat_pos;}
  (junction 6) -> (junction 9) [order 1] : [mka<mk_sat_neg]
  (junction 6) -> (junction 5) [order 2]
  (junction 9) -> (junction 10) : {mki=mki-(1/Tt)*(mka-mk_sat_neg);mka=mk_sat_neg;}
  (junction 10) -> (junction 5)
  (junction 8) -> (junction 10)
  (junction 5) -> (junction 11)
  (junction 11) -> control : {mki_7=mki_6;
      | mki_6=mki_5;
      | mki_5=mki_4;
      | mki_4=mki_3;
      | mki_3=mki_2;
      | mki_2=mki_1;
      | mki_1=mki;
      | ek_6=ek_5; ek_5=ek_4;
      | ek_4=ek_3; ek_3=ek_2;
      | ek_2=ek_1; ek_1=ek;
      | mk=mka}
  data: mkd local double; Tt local double; mk_sat_pos local double; mk_sat_neg local double; ek_1 local double; mki_1 local double; ek local double; mkp local double; mki local double; mk output double; sp input; y input; mka local double; r1 local double; r2 local double; ek_2 local double; mki_2 local double; a0 local double; a1 local double; a2 local double; a3 local double; a4 local double; a5 local double; alfa local double; alfa_lambda local double; lambda_1 local double; mki_3 local double; mki_4 local double; mki_5 local double; mki_6 local double; mki_7 local double; r local double; wc local double; b0 local double; b1 local double; b2 local double; b3 local double; b4 local double; b5 local double; ek_3 local double; ek_4 local double; ek_5 local double; ek_6 local double; alfa_mu local double; kp input double; ki input double; lambda input double; ti local double; td local double; kd input double; mu input double; ts input double

== matlab function FOPIDSOCOptimRand/GCNM/Cost function2/Cost function ==
  settings: updateMethod=DISCRETE
  data: y input; tsf output; time input; ovf output; epsilon input; r input; period input; yTotal input; samplingTime input; refAmplitude input; PmAproxf output
function [tsf,ovf,PmAproxf] = performance(y,time,epsilon,r,period,yTotal,samplingTime,refAmplitude)
        persistent OV tsFlag yHist counter ts PmAprox;
        
        %initialization state
          if isempty(OV)        
              OV=0;
              PmAprox=0;
              tsFlag=1;
              yHist=zeros(1,round(period/(2*samplingTime)));
%               ts=0;
              counter=1;
              ts=0*samplingTime;
              tsf=0;
          end
          
          yHist(counter)=yTotal;
          
          %overshoot and phase margin calculation 
          OVCurrent=(max(y)-refAmplitude);
          tsFlag=max(y);
          if OVCurrent>OV
              OV=OVCurrent;
              ovf=OV;
              OVPor=abs(OV)/refAmplitude+1e-3;     %overshoot percentage
%               OVPor=abs(OV-refAmplitude+0.001)/refAmplitude;     %overshoot percentage
              PmAprox= 100*( -log(OVPor)/ sqrt( pi^2+log(OVPor)^2 )); %approximated phase margin (based on second order system approximation)
              PmAproxf=PmAprox;
          else
              ovf=OV;
              PmAproxf=PmAprox;
          end
          
          %calculate settling time each half of the period
          if mod(time,round(period/2))==0    
            ts=converTimeInv(yHist,10,epsilon);
%             yHist=zeros(1,round(period/2));
            counter=0;
            tsf=ts*samplingTime;
          else
              tsf=ts*samplingTime;
          end
          
          
          if mod(time,period)==0    %restart constraints after each repetitive period
            OV=0;
            PmAprox=0;
          end
          
          counter=counter+1;
          

end
